simulink model "EEDS_model"  (R2015a)
settings: Solver=ode45  StartTime=0.0  StopTime=t_sim  RelTol=1e-3
values from neighbouring files (symbols this model uses):
  B = km*A-F/100    (= -2.59997678)    [EEDS_script.m]
  J = 18.3/(1000*100^2)    (= 1.83e-06)    [EEDS_script.m]
  ke = (V-R*A)    (= 5.88648)    [EEDS_script.m]
  km = (18/1000)/100    (= 0.00018)    [EEDS_script.m]
  L = 331/(10^(-6))    (= 331000000)    [EEDS_script.m]
  R = 0.88    [EEDS_script.m]
libraries: elec_lib x11, fl_lib x6, nesl_utility x5, dspsrcs4 x1
settings Model: Creator=skobr  LastModifiedBy=skobr

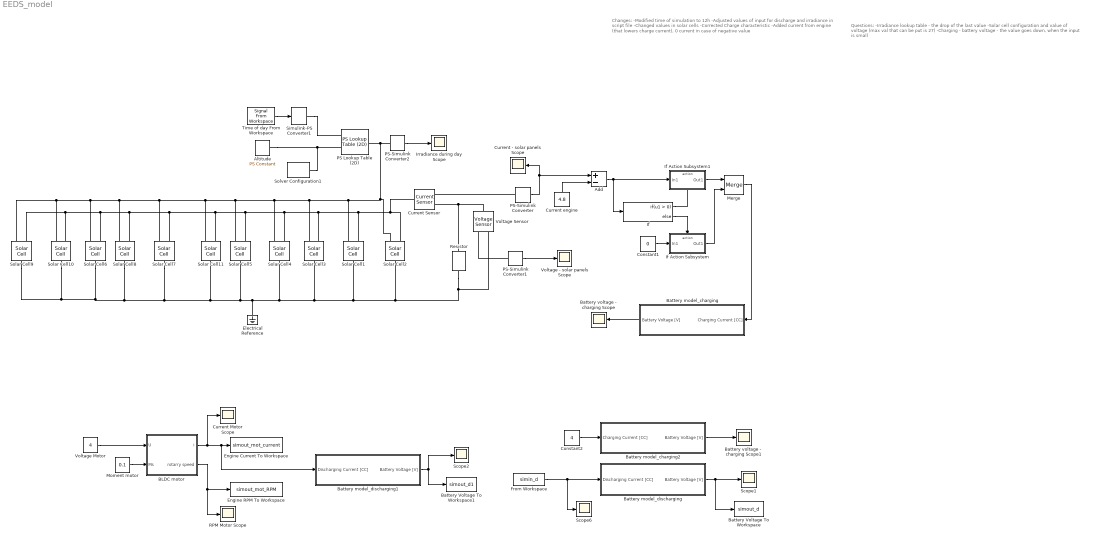
== system EEDS_model ==
  note: Questions:
      | -Irradiance lookup table - the drop of the last value
      | -Solar cell configuration and value of voltage (max val that can be put is 27)
      | -Charging - battery voltage - the value goes down, when the input is small
  note: Changes:
      | -Modified time of simulation to 12h
      | -Adjusted values of input for discharge and irradiance in script file
      | -Changed values in solar cells
      | -Corrected Charge characteristic
      | -Added current from engine (that lowers charge current), 0 current in case of negative value
  Add : Sum  Inputs=+-
  Altitude : fl_lib/Physical Signals/Sources/PS Constant  constant=1000
  BLDC motor : Subsystem
  Battery Voltage To Workspace : ToWorkspace  VariableName=simout_d  SampleTime=-1
  Battery Voltage To Workspace1 : ToWorkspace  VariableName=simout_d1  SampleTime=-1
  Battery model_charging : Subsystem
  Battery model_charging2 : Subsystem
  Battery model_discharging : Subsystem
  Battery model_discharging1 : Subsystem
  Battery voltage -  charging Scope : Scope
      settings: ShowLegends=on  YMin=11  YMax=18  SaveName=ScopeData3
  Battery voltage -  charging Scope1 : Scope
      settings: ShowLegends=on  YMin=14.4  YMax=16.8  SaveName=ScopeData6
  Constant1 : Constant  Value=0
  Constant2 : Constant  Value=4
  Current - solar panels Scope : Scope
      settings: ShowLegends=on  YMin=5.9  YMax=6.8  SaveName=ScopeData4
  Current Motor Scope : Scope
      settings: ShowLegends=on  YMin=4.57531  YMax=5.05693  SaveName=ScopeData8
  Current Sensor : fl_lib/Electrical/Electrical Sensors/Current Sensor
  Current engine : Constant  Value=4.8
  Electrical Reference : fl_lib/Electrical/Electrical Elements/Electrical Reference
  Engine Current To Workspace : ToWorkspace  VariableName=simout_mot_current  SampleTime=-1
  Engine RPM To Workspace : ToWorkspace  VariableName=simout_mot_RPM  SampleTime=-1
  From Workspace : FromWorkspace  VariableName=simin_d  SampleTime=0
  If : If
  If Action Subsystem : Subsystem  TreatAsAtomicUnit=on
  If Action Subsystem1 : Subsystem  TreatAsAtomicUnit=on
  Irradiance during day Scope : Scope
      settings: ShowLegends=on  YMin=0  YMax=2  SaveName=ScopeData2
  Merge : Merge
  Moment motor : Constant  Value=0.1
  PS Lookup Table (2D) : fl_lib/Physical Signals/Lookup Tables/PS Lookup Table (2D)  x_t=[4,5,6,7,8,9,10,11,12,13,14,15,16,17,18,19,20]  y_t=[2000,4000,8000]  z_t=[0,0,0;0,10,90;350,440,600;600,700,900;750,880,1040;820,920,1080;900,980,1100;940,1000,1110;960,1020,1150;940,1000,1140;;900,980,1100;;820,920,1080;750,880,1040;600,700,900;350,440,600;0,10,90;0,0,0]  interp_method=1  extrap_method=1
  PS-Simulink Converter : nesl_utility/PS-Simulink Converter  PhysicalDomain=network_engine_domain  SubClassName=ps_output  LeftPortType=input  RightPortType=output  PseudoPeriodic=off  Frequencies=[]  Unit=1  AffineConversion=off
  PS-Simulink Converter1 : nesl_utility/PS-Simulink Converter  PhysicalDomain=network_engine_domain  SubClassName=ps_output  LeftPortType=input  RightPortType=output  PseudoPeriodic=off  Frequencies=[]  Unit=1  AffineConversion=off
  PS-Simulink Converter2 : nesl_utility/PS-Simulink Converter  PhysicalDomain=network_engine_domain  SubClassName=ps_output  LeftPortType=input  RightPortType=output  PseudoPeriodic=off  Frequencies=[]  Unit=1  AffineConversion=off
  RPM Motor Scope : Scope
      settings: ShowLegends=on  YMin=-0.475494  YMax=-0.475494  SaveName=ScopeData9
  Resistor : fl_lib/Electrical/Electrical Elements/Resistor  R=1 Ohm  i_specify=off  i_priority=High  i=0 A  v_specify=off  v_priority=High  v=0 V
  Scope1 : Scope
      settings: ShowLegends=on  YMin=10  YMax=17
  Scope2 : Scope
      settings: ShowLegends=on  YMin=10  YMax=17  SaveName=ScopeData10
  Scope6 : Scope
      settings: YMin=2  YMax=2  SaveName=ScopeData7
  Simulink-PS Converter1 : nesl_utility/Simulink-PS Converter  PhysicalDomain=network_engine_domain  SubClassName=ps_input  LeftPortType=input  RightPortType=output  PseudoPeriodic=off  Frequencies=[]  NoiseDistribution=none  NoiseParameters=[]  Unit=1  AffineConversion=off  InputFiltering=off  SimscapeFilterOrder=1  InputFilterTimeConstant=0.001  UdotUserProvided=1
  Solar Cell{1..11} (11 alike) : elec_lib/Sources/Solar Cell  prm=1  Isc=0.9 A  Voc=24 V  Is=1e-6 A  Is2=0 A  Iph=7.34 A  Ir0=1000 W/m^2  ec=1.5  N2=2  Rs=0 Ohm  Rp=Inf Ohm  N_series=1  TIPH1=0 1/K  EG=1.11 eV  TXIS1=3  TXIS2=3  TRS1=0  TRP1=0  Tmeas=25 C  TFIXED=25 C  thermal_mass=100 J/K  initial_temperature=25 C
  Solver Configuration1 : nesl_utility/Solver Configuration  PhysicalDomain=network_engine_domain  SubClassName=solver  LeftPortType=input  RightPortType=generic  Accelerate=off  Tones=[]  Harmonics=[]  SimulateNoise=off  Profile=off  UseLocalSampling=off  EnableSwitchedLinearOptims=on  FrequencyDomain=off  UseCCode=off  RelTol=0.001  AbsTol=1e-06  MinStep=1e-09  ToWorkspace=off  RevertToSquareIcSolve=off  NumHomotopyIterations=100  DoDC=off  ResidualTolerance=1e-09  UseLocalSolver=on  LocalSolverChoice=NE_BACKWARD_EULER_ADVANCER  LocalSolverSampleTime=1  DoFixedCost=on  MaxNonlinIter=3  MaxModeIter=2  LinearAlgebra=Sparse  DelaysMemoryBudget=1024  AutomaticFiltering=on  FilteringTimeConstant=0.001
  Time of day From Workspace : dspsrcs4/Signal From Workspace  X=irr_time  Ts=1  nsamps=1  OutputAfterFinalValue=Setting to zero  ignoreOrWarnInputAndFrameLengths=off
  Voltage - solar panels Scope : Scope
      settings: ShowLegends=on  YMin=0  YMax=2  SaveName=ScopeData5
  Voltage Motor : Constant  Value=4
  Voltage Sensor : fl_lib/Electrical/Electrical Sensors/Voltage Sensor
  wires:
  Battery model_discharging/1(Battery Voltage [V]) -> Battery Voltage To Workspace/1, Scope1/1
  Battery model_charging/1(Battery Voltage [V]) -> Battery voltage -  charging Scope/1
  From Workspace/1 -> Scope6/1, Battery model_discharging/1(Discharging Current [CC])
  PS-Simulink Converter1/1 -> Voltage - solar panels Scope/1
  PS-Simulink Converter2/1 -> Irradiance during day Scope/1
  Time of day From Workspace/1 -> Simulink-PS Converter1/1
  PS-Simulink Converter/1 -> Current - solar panels Scope/1, Add/1
  Current engine/1 -> Add/2
  Add/1 -> If/1, If Action Subsystem1/1(In1)
  If/1 -> If Action Subsystem1/Action
  If/2 -> If Action Subsystem/Action
  If Action Subsystem/1(Out1) -> Merge/2
  Constant1/1 -> If Action Subsystem/1(In1)
  If Action Subsystem1/1(Out1) -> Merge/1
  Merge/1 -> Battery model_charging/1(Charging Current [CC])
  Battery model_charging2/1(Battery Voltage [V]) -> Battery voltage -  charging Scope1/1
  Constant2/1 -> Battery model_charging2/1(Charging Current [CC])
  Voltage Motor/1 -> BLDC motor/1("U ")
  Moment motor/1 -> BLDC motor/2(Ms)
  BLDC motor/2(rotarry speed) -> RPM Motor Scope/1, Engine RPM To Workspace/1
  Battery model_discharging1/1(Battery Voltage [V]) -> Scope2/1, Battery Voltage To Workspace1/1
  BLDC motor/1(i) -> Battery model_discharging1/1(Discharging Current [CC]), Engine Current To Workspace/1, Current Motor Scope/1
  connections:
  Voltage Sensor/LConn1 -- Resistor/LConn1 -- Current Sensor/RConn2
  Electrical Reference/LConn1 -- Solar Cell5/RConn1 -- Solar Cell7/RConn1 -- Solar Cell9/RConn1 -- Solar Cell10/RConn1 -- Solar Cell6/RConn1 -- Solar Cell8/RConn1 -- Solar Cell11/RConn1 -- Solar Cell4/RConn1 -- Solar Cell3/RConn1 -- Solar Cell1/RConn1 -- Solar Cell2/RConn1 -- Resistor/RConn1 -- Voltage Sensor/RConn2
  PS-Simulink Converter1/LConn1 -- Voltage Sensor/RConn1
  PS-Simulink Converter/LConn1 -- Current Sensor/RConn1
  Solar Cell2/LConn2 -- Solar Cell9/LConn2 -- Solar Cell10/LConn2 -- Solar Cell6/LConn2 -- Solar Cell8/LConn2 -- Solar Cell7/LConn2 -- Solar Cell11/LConn2 -- Solar Cell5/LConn2 -- Solar Cell4/LConn2 -- Solar Cell3/LConn2 -- Solar Cell1/LConn2 -- Current Sensor/LConn1
  Simulink-PS Converter1/RConn1 -- PS Lookup Table (2D)/LConn1
  Altitude/RConn1 -- Solver Configuration1/RConn1 -- PS Lookup Table (2D)/LConn2
  Solar Cell9/LConn1 -- Solar Cell10/LConn1 -- Solar Cell6/LConn1 -- Solar Cell8/LConn1 -- Solar Cell7/LConn1 -- Solar Cell11/LConn1 -- Solar Cell5/LConn1 -- Solar Cell4/LConn1 -- Solar Cell3/LConn1 -- Solar Cell1/LConn1 -- Solar Cell2/LConn1 -- PS Lookup Table (2D)/RConn1 -- PS-Simulink Converter2/LConn1

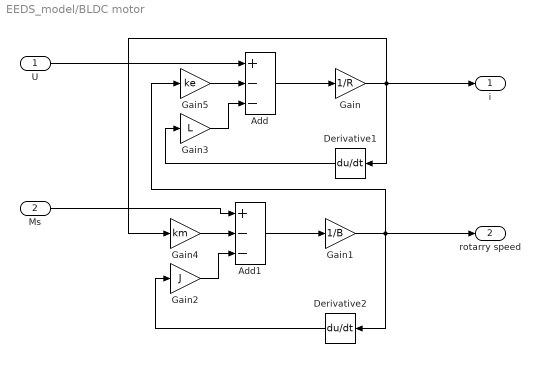
== system EEDS_model/BLDC motor ==
  "U " : Inport
  Ms : Inport  Port=2
  Add : Sum  Inputs=+--
  Add1 : Sum  Inputs=+--
  Derivative1 : Derivative
  Derivative2 : Derivative
  Gain : Gain  Gain=1/R
  Gain1 : Gain  Gain=1/B
  Gain2 : Gain  Gain=J
  Gain3 : Gain  Gain=L
  Gain4 : Gain  Gain=km
  Gain5 : Gain  Gain=ke
  i : Outport
  rotarry speed : Outport  Port=2
  wires:
  Derivative2/1 -> Gain2/1
  Gain1/1 -> rotarry speed/1, Derivative2/1, Gain5/1
  Gain4/1 -> Add1/2
  Add/1 -> Gain/1
  Gain2/1 -> Add1/3
  Derivative1/1 -> Gain3/1
  Ms/1 -> Add1/1
  Add1/1 -> Gain1/1
  Gain/1 -> i/1, Derivative1/1, Gain4/1
  "U "/1 -> Add/1
  Gain3/1 -> Add/3
  Gain5/1 -> Add/2

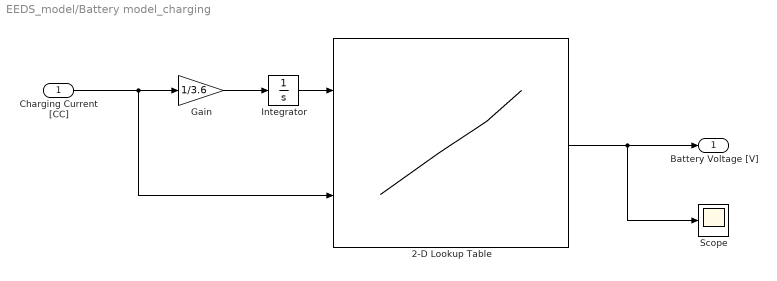
== system EEDS_model/Battery model_charging ==
  Charging Current [CC] : Inport
  2-D Lookup Table : Lookup_n-D  BreakpointsForDimension1=16*3300*[0,0.1,0.2,0.3,0.4,0.5,0.6,0.7,0.8,0.9,0.95,1]  BreakpointsForDimension2=[1,2]  Table=reshape(4*[3,3.45,3.6,3.65,3.7,3.75,3.8,3.87,3.95,4.08,4.2,4.2,3,3.6,3.8,3.85,3.87,3.9,3.93,3.97,4.05,4.2,4.2,4.2],12,2)  InternalRulePriority=Speed  RndMeth=Simplest  InputSameDT=on
  Gain : Gain  Gain=1/3.6
  Integrator : Integrator
  Scope : Scope
      settings: YMin=-7.4125  YMax=5.49028
  Battery Voltage [V] : Outport
  wires:
  2-D Lookup Table/1 -> Battery Voltage [V]/1, Scope/1
  Charging Current [CC]/1 -> 2-D Lookup Table/2, Gain/1
  Integrator/1 -> 2-D Lookup Table/1
  Gain/1 -> Integrator/1

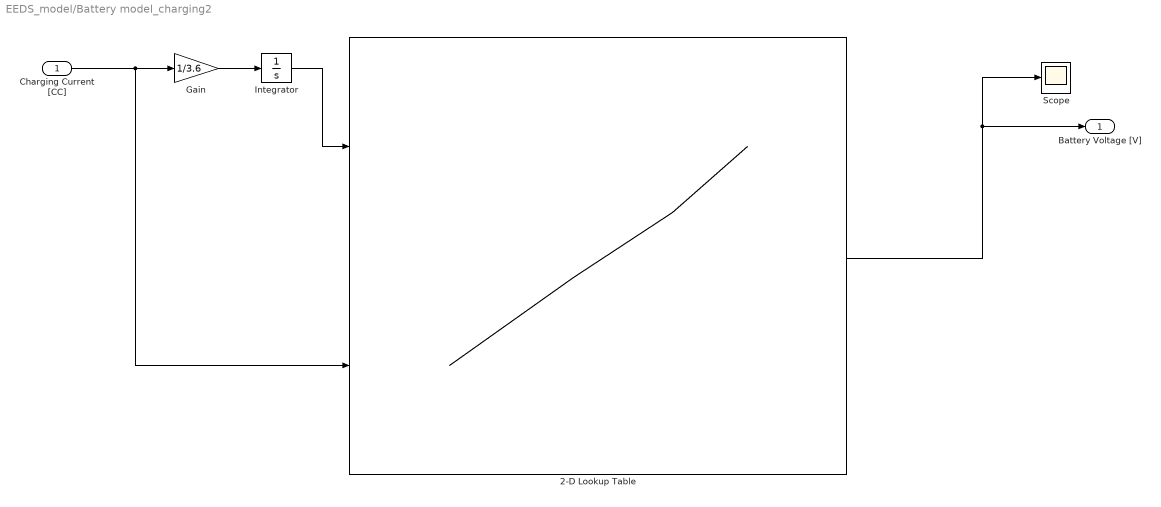
== system EEDS_model/Battery model_charging2 ==
  Charging Current [CC] : Inport
  2-D Lookup Table : Lookup_n-D  BreakpointsForDimension1=16*3300*[0,0.1,0.2,0.3,0.4,0.5,0.6,0.7,0.8,0.9,0.95,1]  BreakpointsForDimension2=[1,2]  Table=reshape(4*[3,3.45,3.6,3.65,3.7,3.75,3.8,3.87,3.95,4.08,4.2,4.2,3,3.6,3.8,3.85,3.87,3.9,3.93,4.0,4.05,4.2,4.2,4.2],12,2)  InternalRulePriority=Speed  RndMeth=Simplest  InputSameDT=on
  Gain : Gain  Gain=1/3.6
  Integrator : Integrator
  Scope : Scope
      settings: YMin=-7.4125  YMax=5.49028
  Battery Voltage [V] : Outport
  wires:
  2-D Lookup Table/1 -> Scope/1, Battery Voltage [V]/1
  Charging Current [CC]/1 -> 2-D Lookup Table/2, Gain/1
  Integrator/1 -> 2-D Lookup Table/1
  Gain/1 -> Integrator/1

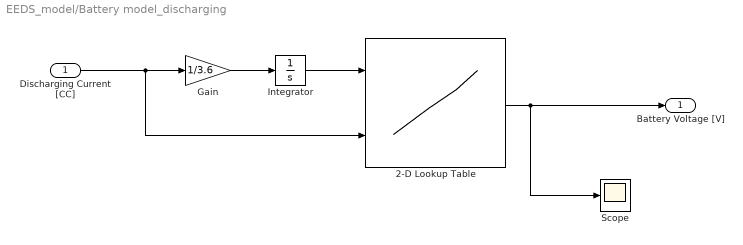
== system EEDS_model/Battery model_discharging ==
  Discharging Current [CC] : Inport
  2-D Lookup Table : Lookup_n-D  BreakpointsForDimension1=16*[0,50,100,200,2900,3000,3100,3200,3300,3400]  BreakpointsForDimension2=[0,0.2,0.5,1,2]  Table=reshape(4*[4.2,4.12,4.1,4.04,3.32,3.28,3.25,3.12,3.0,2.5,4.2,4.12,4.1,4.04,3.32,3.28,3.25,3.12,3.0,2.5,4.2,4.05,4,3.95,3.19,3.15,3.05,2.85,2.5,2.5,4.2,3.95,3.9,3.84,3.0,2.92,2.85,2.65,2.5,2.5,4.2,3.8,3.72,3.65,2.8,2.75,2.7,2.61,2.5,2.5],10,5)  InternalRulePriority=Speed  RndMeth=Simplest  InputSameDT=on
  Gain : Gain  Gain=1/3.6
  Integrator : Integrator
  Scope : Scope
      settings: YMin=-7.4125  YMax=5.49028
  Battery Voltage [V] : Outport
  wires:
  2-D Lookup Table/1 -> Scope/1, Battery Voltage [V]/1
  Discharging Current [CC]/1 -> 2-D Lookup Table/2, Gain/1
  Integrator/1 -> 2-D Lookup Table/1
  Gain/1 -> Integrator/1

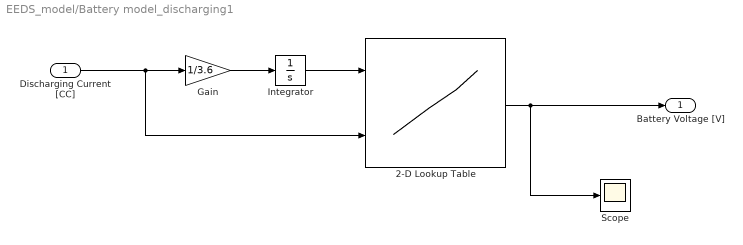
== system EEDS_model/Battery model_discharging1 ==
  Discharging Current [CC] : Inport
  2-D Lookup Table : Lookup_n-D  BreakpointsForDimension1=16*[0,50,100,200,2900,3000,3100,3200,3300,3400]  BreakpointsForDimension2=[0,0.2,0.5,1,2]  Table=reshape(4*[4.2,4.12,4.1,4.04,3.32,3.28,3.25,3.12,3.0,2.5,4.2,4.12,4.1,4.04,3.32,3.28,3.25,3.12,3.0,2.5,4.2,4.05,4,3.95,3.19,3.15,3.05,2.85,2.5,2.5,4.2,3.95,3.9,3.84,3.0,2.92,2.85,2.65,2.5,2.5,4.2,3.8,3.72,3.65,2.8,2.75,2.7,2.61,2.5,2.5],10,5)  InternalRulePriority=Speed  RndMeth=Simplest  InputSameDT=on
  Gain : Gain  Gain=1/3.6
  Integrator : Integrator
  Scope : Scope
      settings: YMin=-7.4125  YMax=5.49028
  Battery Voltage [V] : Outport
  wires:
  2-D Lookup Table/1 -> Scope/1, Battery Voltage [V]/1
  Discharging Current [CC]/1 -> 2-D Lookup Table/2, Gain/1
  Integrator/1 -> 2-D Lookup Table/1
  Gain/1 -> Integrator/1

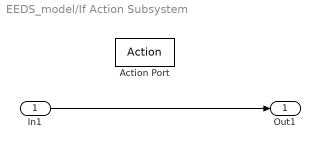
== system EEDS_model/If Action Subsystem ==
  In1 : Inport
  Action Port : ActionPort  ActionType=else
  Out1 : Outport
  wires:
  In1/1 -> Out1/1

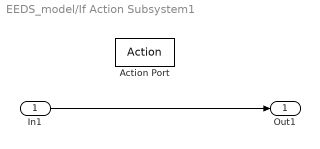
== system EEDS_model/If Action Subsystem1 ==
  In1 : Inport
  Action Port : ActionPort  ActionType=then
  Out1 : Outport
  wires:
  In1/1 -> Out1/1
